simulink model "player_ball_7_8players2"  (R2021b)
settings: Solver=VariableStepAuto  StartTime=0.0  StopTime=300  RelTol=1e-3
model workspace (MAT data in the model file):
  trailfuzzy = 'trailfuzzy.fis'
values from neighbouring files (symbols this model uses):
  initBallPos = fieldCenter    [robotSoccerParams.m]
  robotDetectorMaxHits = 5    [robotSoccerParams.m]
  sampleTime = 0.05    [robotSoccerParams.m]
undefined symbols (not defined in the file or in its folder): DiscIntNeverNeededParam
libraries: mobileRoboticsLib x41, dspindex x13, fuzblock x8
(part 1 of 2)
settings Model: NumberOfSteps=10  Creator=kstkr  LastModifiedBy=kstkr
settings DebuggingCC: AlgebraicLoopMsg=none

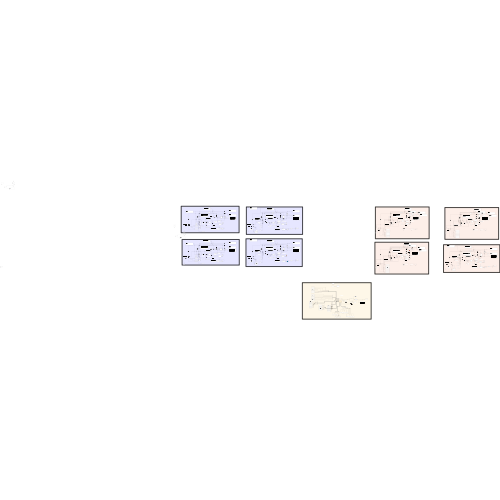
[thumbnail: Simulink's stored preview of the top-level diagram]
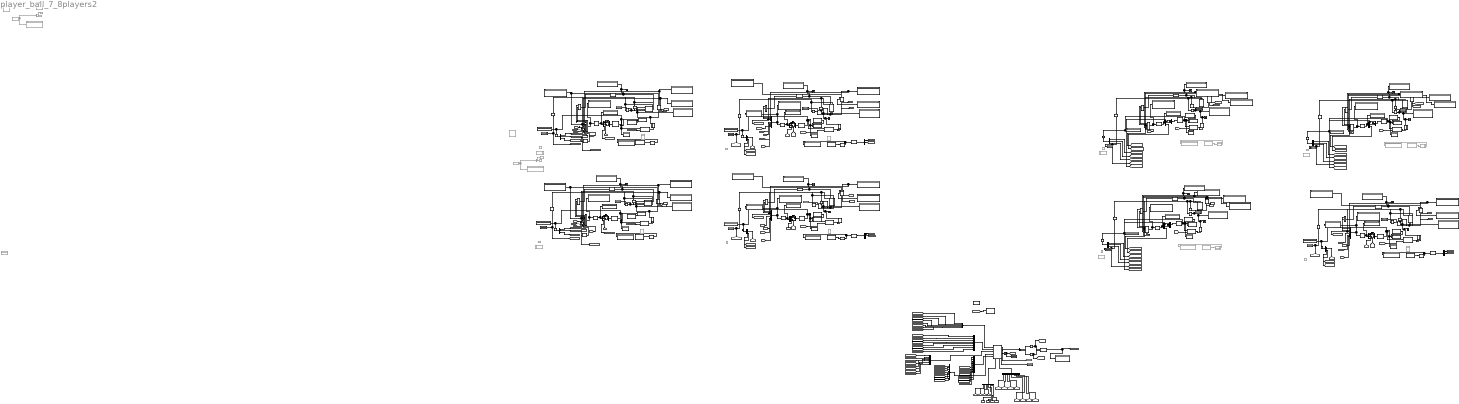
== system player_ball_7_8players2 ==
  note: Subsystem1
  note: Subsystem1
  note: Ensure the sensor parameters point to the same variables.
  note: Checks team possession and ball held
  note: change mf to sinesoidal
  note: check for postition 80,10
  note: Subsystem1
  note: change mf to sinesoidal
  note: check for postition 80,10
  note: Subsystem1
  note: Ensure the sensor parameters point to the same variables.
  note: Subsystem1
  note: Ensure the sensor parameters point to the same variables.
  note: Subsystem1
  note: Ensure the sensor parameters point to the same variables.
  note: Subsystem1
  note: Ensure the sensor parameters point to the same variables.
  note: Subsystem1
  note: Ensure the sensor parameters point to the same variables.
  Add Constant{,1..3} (4 alike) : Bias  Commented=on  Bias=0.3
  Ball Dynamics : MATLAB Function  Commented=on  TreatAsAtomicUnit=on
  Ball Dynamics1 : MATLAB Function  Commented=on  TreatAsAtomicUnit=on
  Ball Dynamics2 : MATLAB Function  Commented=on  TreatAsAtomicUnit=on
  Ball Dynamics3 : MATLAB Function  Commented=on  TreatAsAtomicUnit=on
  Ball Dynamics4 : MATLAB Function  Commented=on  TreatAsAtomicUnit=on
  Ball Dynamics5 : MATLAB Function  Commented=on  TreatAsAtomicUnit=on
  Ball Dynamics6 : MATLAB Function  Commented=on  TreatAsAtomicUnit=on
  Bus Creator{,1..6} (7 alike) : BusCreator  Inputs=8
  Chart3 : Stateflow chart  TreatAsAtomicUnit=on
      settings: PortSchema="{\"entries\":[{\"content\":{\"sides\":[{\"content\":{\"connectorIds\":[\"In1\",\"In2\",\"In3\",\"In4\",\"In6\"]},\"type\":\"ConnectorPlacement.EquallySpacedRectSide\",\"uuid\":\"100227f9-96df-4219-ace2-0d84d12d506e\"},{\"content\":{\"connectorIds\":[\"Out1\",\"Out2\",\"Out3\",\"Out4\"],\"side\":\"RIGHT\"},\"type\":\"ConnectorPlacement.EquallySpacedRectSide\",\"uuid\":\"5179a9f1-5caf-4bf7-8381-53191773d399\"},{\"content\":{\"connectorIds\":[],\"side\":\"TOP\"},\"type\":\"ConnectorPlacement.EquallySpacedRectSide\",\"uuid\":\"b02881a3-df96-4ac6-93d3-ffe2a0056366\"},{\"content\":{\"connectorIds\":[\"In7\",\"In5\"],\"side\":\"BOTTOM\"},\"type\":\"ConnectorPlacement.EquallySpacedRectSide\",\"uuid\":\"6df5f698-3dd3-4c11-801f-bca33302808b\"}]},\"type\":\"ConnectorPlacement.EquallySpacedConnector\",\"uuid\":\"a5fc3484-c51e-4d4d-931a-fb20b747c02a\"}],\"packageUris\":[\"http://schema.mathworks.com/mf0/Connector/R2020b\"],\"version\":\"1.0\"}"
  Constant{,1..8} (9 alike) : Constant  Commented=on  Value=0.5
  Demux{,1..3,5..10,12..24,26..29} (27 alike) : Demux  Outputs=3
  Demux11 : Demux  Outputs=2
  Demux25 : Demux  Commented=on  Outputs=2
  Demux4 : Demux  Commented=on  Outputs=2
  Display{,1..9,11..41,43..49,51..58,60..69,71..84,86..87} (82 alike) : Display
  Display{10,42,50,59,70} (5 alike) : Display  Commented=on
  Generic Vehicle Simulation : mobileRoboticsLib/Utilities/Generic Vehicle Simulation  initX=40  initY=10  initAngle=0  Ts=sampleTime
      settings: SourceProductName=Mobile Robotics Simulation Toolbox
  Generic Vehicle Simulation1 : mobileRoboticsLib/Utilities/Generic Vehicle Simulation  initX=30  initY=50  initAngle=0  Ts=sampleTime
      settings: SourceProductName=Mobile Robotics Simulation Toolbox
  Generic Vehicle Simulation2 : mobileRoboticsLib/Utilities/Generic Vehicle Simulation  initX=25  initY=30  initAngle=0  Ts=sampleTime
      settings: SourceProductName=Mobile Robotics Simulation Toolbox
  Generic Vehicle Simulation3 : mobileRoboticsLib/Utilities/Generic Vehicle Simulation  initX=2  initY=30  initAngle=0  Ts=sampleTime
      settings: SourceProductName=Mobile Robotics Simulation Toolbox
  Generic Vehicle Simulation4 : mobileRoboticsLib/Utilities/Generic Vehicle Simulation  initX=60  initY=40  initAngle=pi  Ts=sampleTime
      settings: SourceProductName=Mobile Robotics Simulation Library
  Generic Vehicle Simulation5 : mobileRoboticsLib/Utilities/Generic Vehicle Simulation  initX=60  initY=20  initAngle=pi  Ts=sampleTime
      settings: SourceProductName=Mobile Robotics Simulation Library
  Generic Vehicle Simulation6 : mobileRoboticsLib/Utilities/Generic Vehicle Simulation  initX=75  initY=30  initAngle=pi  Ts=sampleTime
      settings: SourceProductName=Mobile Robotics Simulation Library
  Generic Vehicle Simulation7 : mobileRoboticsLib/Utilities/Generic Vehicle Simulation  initX=88  initY=30  initAngle=pi  Ts=sampleTime
      settings: SourceProductName=Mobile Robotics Simulation Toolbox
  Goal Range{,1..4} (5 alike) : Display
  GoalLeftAngle{,1..4} (5 alike) : Display
  Ground{,1..7} (8 alike) : Ground
  IC{1,4,7,10,13,16,19,22} (8 alike) : InitialCondition
  IC{2..3,5..6,8..9,11..12,14..15,17..18,20..21,23..24} (16 alike) : InitialCondition  Value=0
  MATLAB Function : MATLAB Function  TreatAsAtomicUnit=on
  MATLAB Function1 : MATLAB Function  TreatAsAtomicUnit=on
  Memory{,2..4,7..10} (8 alike) : Memory  InitialCondition=[15 2 0]  InheritSampleTime=on
  Memory1 : Memory  InheritSampleTime=on
  Memory5 : Memory  InheritSampleTime=on  LinearizeAsDelay=on
  Memory6 : Memory  InheritSampleTime=on  LinearizeAsDelay=on
  Multi-Robot Environment : mobileRoboticsLib/Environments/Multi-Robot Environment  numRobots=8  mapName=map  showWaypoints=off  showObjects=on  objectColors=objColors  objectMarkers=objMarkers  showRobotIds=on  plotSensorLines=on
      settings: SourceProductName=Mobile Robotics Simulation Toolbox
  Multi-Robot Lidar Sensor1 : mobileRoboticsLib/Environments/Multi-Robot Lidar Sensor  robotIdx=1  mapName=map  sensorOffset=[0,0]  scanAngles=[-pi/4 0 pi/4]  maxRange=5
      settings: SourceProductName=Mobile Robotics Simulation Toolbox
  Multi-Robot Lidar Sensor2 : mobileRoboticsLib/Environments/Multi-Robot Lidar Sensor  robotIdx=2  mapName=map  sensorOffset=[0,0]  scanAngles=[-pi/4 0 pi/4]  maxRange=5
      settings: SourceProductName=Mobile Robotics Simulation Toolbox
  Multi-Robot Lidar Sensor3 : mobileRoboticsLib/Environments/Multi-Robot Lidar Sensor  robotIdx=3  mapName=map  sensorOffset=[0,0]  scanAngles=[-pi/4 0 pi/4]  maxRange=5
      settings: SourceProductName=Mobile Robotics Simulation Toolbox
  Multi-Robot Lidar Sensor4 : mobileRoboticsLib/Environments/Multi-Robot Lidar Sensor  robotIdx=4  mapName=map  sensorOffset=[0,0]  scanAngles=[-pi/4 0 pi/4]  maxRange=5
      settings: SourceProductName=Mobile Robotics Simulation Toolbox
  Multi-Robot Lidar Sensor5 : mobileRoboticsLib/Environments/Multi-Robot Lidar Sensor  robotIdx=5  mapName=map  sensorOffset=[0,0]  scanAngles=[-pi/4 0 pi/4]  maxRange=5
      settings: SourceProductName=Mobile Robotics Simulation Toolbox
  Multi-Robot Lidar Sensor6 : mobileRoboticsLib/Environments/Multi-Robot Lidar Sensor  robotIdx=6  mapName=map  sensorOffset=[0,0]  scanAngles=[-pi/4 0 pi/4]  maxRange=5
      settings: SourceProductName=Mobile Robotics Simulation Toolbox
  Multi-Robot Lidar Sensor7 : mobileRoboticsLib/Environments/Multi-Robot Lidar Sensor  robotIdx=7  mapName=map  sensorOffset=[0,0]  scanAngles=[-pi/4 0 pi/4]  maxRange=5
      settings: SourceProductName=Mobile Robotics Simulation Toolbox
  Multi-Robot Lidar Sensor8 : mobileRoboticsLib/Environments/Multi-Robot Lidar Sensor  robotIdx=8  mapName=map  sensorOffset=[0,0]  scanAngles=[-pi/4 0 pi/4]  maxRange=5
      settings: SourceProductName=Mobile Robotics Simulation Toolbox
  Multi-Robot Visualizer : mobileRoboticsLib/Environments/Multi-Robot Visualizer  idx=1  radius=1  robotColor=[0 0 1]  showTraj=on  hasLidar=on  sensorOffset=[0,0]  scanAngles=[-pi/4 0 pi/4]  maxNumScans=0  hasObjDetector=off  objDetectorOffset=[0,0]  objDetectorAngle=0  objDetectorFOV=pi/3  objDetectorMaxRange=5  hasRobotDetector=off  robotDetectorOffset=[0,0]  robotDetectorAngle=0  robotDetectorFOV=pi/3  robotDetectorMaxRange=5  robotDetectorNumDetections=0
      settings: SourceProductName=Mobile Robotics Simulation Toolbox
  Multi-Robot Visualizer1 : mobileRoboticsLib/Environments/Multi-Robot Visualizer  idx=3  radius=1  robotColor=[0 0 1]  showTraj=on  hasLidar=on  sensorOffset=[0,0]  scanAngles=[-pi/4 0 pi/4]  maxNumScans=0  hasObjDetector=off  objDetectorOffset=[0,0]  objDetectorAngle=0  objDetectorFOV=pi/3  objDetectorMaxRange=5  hasRobotDetector=off  robotDetectorOffset=[0,0]  robotDetectorAngle=0  robotDetectorFOV=pi/3  robotDetectorMaxRange=5  robotDetectorNumDetections=0
      settings: SourceProductName=Mobile Robotics Simulation Toolbox
  Multi-Robot Visualizer2 : mobileRoboticsLib/Environments/Multi-Robot Visualizer  idx=2  radius=1  robotColor=[0 0 1]  showTraj=on  hasLidar=on  sensorOffset=[0,0]  scanAngles=[-pi/4 0 pi/4]  maxNumScans=0  hasObjDetector=off  objDetectorOffset=[0,0]  objDetectorAngle=0  objDetectorFOV=pi/3  objDetectorMaxRange=5  hasRobotDetector=off  robotDetectorOffset=[0,0]  robotDetectorAngle=0  robotDetectorFOV=pi/3  robotDetectorMaxRange=5  robotDetectorNumDetections=0
      settings: SourceProductName=Mobile Robotics Simulation Toolbox
  Multi-Robot Visualizer3 : mobileRoboticsLib/Environments/Multi-Robot Visualizer  idx=4  radius=1  robotColor=[0 0 1]  showTraj=on  hasLidar=on  sensorOffset=[0,0]  scanAngles=[-pi/4 0 pi/4]  maxNumScans=0  hasObjDetector=off  objDetectorOffset=[0,0]  objDetectorAngle=0  objDetectorFOV=pi/3  objDetectorMaxRange=5  hasRobotDetector=off  robotDetectorOffset=[0,0]  robotDetectorAngle=0  robotDetectorFOV=pi/3  robotDetectorMaxRange=5  robotDetectorNumDetections=0
      settings: SourceProductName=Mobile Robotics Simulation Toolbox
  Multi-Robot Visualizer4 : mobileRoboticsLib/Environments/Multi-Robot Visualizer  idx=5  radius=1  robotColor=[1 0 0]  showTraj=on  hasLidar=on  sensorOffset=[0,0]  scanAngles=[-pi/4 0 pi/4]  maxNumScans=0  hasObjDetector=off  objDetectorOffset=[0,0]  objDetectorAngle=0  objDetectorFOV=pi/3  objDetectorMaxRange=5  hasRobotDetector=off  robotDetectorOffset=[0,0]  robotDetectorAngle=0  robotDetectorFOV=pi/3  robotDetectorMaxRange=5  robotDetectorNumDetections=0
      settings: SourceProductName=Mobile Robotics Simulation Toolbox
  Multi-Robot Visualizer5 : mobileRoboticsLib/Environments/Multi-Robot Visualizer  idx=6  radius=1  robotColor=[1 0 0]  showTraj=on  hasLidar=on  sensorOffset=[0,0]  scanAngles=[-pi/4 0 pi/4]  maxNumScans=0  hasObjDetector=off  objDetectorOffset=[0,0]  objDetectorAngle=0  objDetectorFOV=pi/3  objDetectorMaxRange=5  hasRobotDetector=off  robotDetectorOffset=[0,0]  robotDetectorAngle=0  robotDetectorFOV=pi/3  robotDetectorMaxRange=5  robotDetectorNumDetections=0
      settings: SourceProductName=Mobile Robotics Simulation Toolbox
  Multi-Robot Visualizer6 : mobileRoboticsLib/Environments/Multi-Robot Visualizer  idx=7  radius=1  robotColor=[1 0 0]  showTraj=on  hasLidar=on  sensorOffset=[0,0]  scanAngles=[-pi/4 0 pi/4]  maxNumScans=0  hasObjDetector=off  objDetectorOffset=[0,0]  objDetectorAngle=0  objDetectorFOV=pi/3  objDetectorMaxRange=5  hasRobotDetector=off  robotDetectorOffset=[0,0]  robotDetectorAngle=0  robotDetectorFOV=pi/3  robotDetectorMaxRange=5  robotDetectorNumDetections=0
      settings: SourceProductName=Mobile Robotics Simulation Toolbox
  Multi-Robot Visualizer7 : mobileRoboticsLib/Environments/Multi-Robot Visualizer  idx=8  radius=1  robotColor=[1 0 0]  showTraj=on  hasLidar=on  sensorOffset=[0,0]  scanAngles=[-pi/4 0 pi/4]  maxNumScans=0  hasObjDetector=off  objDetectorOffset=[0,0]  objDetectorAngle=0  objDetectorFOV=pi/3  objDetectorMaxRange=5  hasRobotDetector=off  robotDetectorOffset=[0,0]  robotDetectorAngle=0  robotDetectorFOV=pi/3  robotDetectorMaxRange=5  robotDetectorNumDetections=0
      settings: SourceProductName=Mobile Robotics Simulation Toolbox
  Mux{,1,4,6,8,10,12,14} (8 alike) : Mux  Inputs=3
  Mux11 : Mux  Inputs=7
  Mux13 : Mux  Inputs=7
  Mux15 : Mux  Inputs=8
  Mux2 : Mux  Inputs=11
  Mux3 : Mux  Inputs=11
  Mux5 : Mux  Inputs=9
  Mux7 : Mux  Inputs=8
  Mux9 : Mux  Inputs=7
  Object Detections [range, angle, label]{,1..7} (8 alike) : Display
  Object Detector{,1..7} (8 alike) : mobileRoboticsLib/Environments/Object Detector  mapName=map  sensorOffset=objDetectorOffset  sensorAngle=objDetectorAngle  fieldOfView=objDetectorFOV  maxRange=objDetectorRange  maxDetections=objDetectorMaxHits  sampleTime=-1
      Object Detector settings: SourceProductName=Mobile Robotics Simulation Toolbox
      Object Detector1 settings: SourceProductName=Mobile Robotics Simulation Toolbox
      Object Detector2 settings: SourceProductName=Mobile Robotics Simulation Toolbox
      Object Detector3 settings: SourceProductName=Mobile Robotics Simulation Toolbox
      Object Detector4 settings: SourceProductName=Ground Vehicles Library
      Object Detector5 settings: SourceProductName=Ground Vehicles Library
      Object Detector6 settings: SourceProductName=Ground Vehicles Library
      Object Detector7 settings: SourceProductName=Mobile Robotics Simulation Toolbox
  "Objects [x, y, label]1" : Constant  Commented=on  Value=[45, 30, 1; 0,15,2; 0, 45, 2; 90, 15, 3; 90, 45, 3]
  "Objects [x, y, label]2" : Constant  Commented=on  Value=[45, 30, 1; 0,15,2; 0, 45, 2; 90, 15, 3; 90, 45, 3]
  Package Objects Array1 : Subsystem
  Plot Soccer Field : MATLAB Function  TreatAsAtomicUnit=on
  Robot Detector1 : mobileRoboticsLib/Environments/Robot Detector  mapName=map  robotIdx=1  sensorOffset=robotDetectorOffset  sensorAngle=robotDetectorAngle  sensorFOV=2*pi  maxRange=100  maxDetections=robotDetectorMaxHits  sampleTime=sampleTime
      link override Robot Detector: mapName=map  maxDetections=5
      settings: SourceProductName=Mobile Robotics Simulation Toolbox
  Robot Detector2 : mobileRoboticsLib/Environments/Robot Detector  mapName=map  robotIdx=2  sensorOffset=robotDetectorOffset  sensorAngle=robotDetectorAngle  sensorFOV=2*pi  maxRange=100  maxDetections=robotDetectorMaxHits  sampleTime=sampleTime
      link override Robot Detector: mapName=map  maxDetections=5
      settings: SourceProductName=Mobile Robotics Simulation Toolbox
  Robot Detector3 : mobileRoboticsLib/Environments/Robot Detector  mapName=map  robotIdx=3  sensorOffset=robotDetectorOffset  sensorAngle=robotDetectorAngle  sensorFOV=2*pi  maxRange=100  maxDetections=robotDetectorMaxHits  sampleTime=sampleTime
      link override Robot Detector: mapName=map  maxDetections=5
      settings: SourceProductName=Mobile Robotics Simulation Toolbox
  Robot Detector4 : mobileRoboticsLib/Environments/Robot Detector  mapName=map  robotIdx=4  sensorOffset=robotDetectorOffset  sensorAngle=robotDetectorAngle  sensorFOV=2*pi  maxRange=100  maxDetections=robotDetectorMaxHits  sampleTime=sampleTime
      link override Robot Detector: mapName=map  maxDetections=5
      settings: SourceProductName=Mobile Robotics Simulation Toolbox
  Robot Detector5 : mobileRoboticsLib/Environments/Robot Detector  Commented=on  mapName=map  robotIdx=1  sensorOffset=robotDetectorOffset  sensorAngle=robotDetectorAngle  sensorFOV=pi/3  maxRange=100  maxDetections=robotDetectorMaxHits  sampleTime=sampleTime
      link override Robot Detector: mapName=map  maxDetections=5
      settings: SourceProductName=Mobile Robotics Simulation Toolbox
  Robot Detector6 : mobileRoboticsLib/Environments/Robot Detector  Commented=on  mapName=map  robotIdx=1  sensorOffset=robotDetectorOffset  sensorAngle=robotDetectorAngle  sensorFOV=pi/3  maxRange=100  maxDetections=robotDetectorMaxHits  sampleTime=sampleTime
      link override Robot Detector: mapName=map  maxDetections=5
      settings: SourceProductName=Mobile Robotics Simulation Toolbox
  Robot Detector7 : mobileRoboticsLib/Environments/Robot Detector  Commented=on  mapName=map  robotIdx=1  sensorOffset=robotDetectorOffset  sensorAngle=robotDetectorAngle  sensorFOV=pi/3  maxRange=100  maxDetections=robotDetectorMaxHits  sampleTime=sampleTime
      link override Robot Detector: mapName=map  maxDetections=5
      settings: SourceProductName=Mobile Robotics Simulation Toolbox
  Robot Detector8 : mobileRoboticsLib/Environments/Robot Detector  mapName=map  robotIdx=8  sensorOffset=robotDetectorOffset  sensorAngle=robotDetectorAngle  sensorFOV=2*pi  maxRange=100  maxDetections=robotDetectorMaxHits  sampleTime=sampleTime
      link override Robot Detector: mapName=map  maxDetections=5
      settings: SourceProductName=Mobile Robotics Simulation Toolbox
  Scope{,1..2,4,6,8,10,12} (8 alike) : Scope
  Scope{3,5,7,9,11,13} (6 alike) : Scope  NumInputPorts=2
  Variable Selector{,1,3..8,10..12} (11 alike) : dspindex/Variable Selector  NumInputs=1  rowsOrCols=Rows  IdxMode=Fixed  Elements="[1  ]"  ZerOneIdxMode=One-based  errmode=Clip Index  FillMode=off  FillValues=0
  Variable Selector2 : dspindex/Variable Selector  Commented=on  NumInputs=1  rowsOrCols=Columns  IdxMode=Fixed  Elements=[1 2]  ZerOneIdxMode=One-based  errmode=Clip Index  FillMode=on  FillValues=0
  Variable Selector9 : dspindex/Variable Selector  Commented=on  NumInputs=1  rowsOrCols=Columns  IdxMode=Fixed  Elements=[1 2]  ZerOneIdxMode=One-based  errmode=Clip Index  FillMode=on  FillValues=0
  Zero Pad Detections1 : MATLAB Function  TreatAsAtomicUnit=on  mask(Zero Pad Detections){maxHits=robotDetectorMaxHits}
      mask prompts: maxHits "Maximum Sensor Hits"
      mask help: Zero pads detections matrix so it is fixed-size and works with arrays of buses.
  Zero Pad Detections10 : MATLAB Function  TreatAsAtomicUnit=on  mask(Zero Pad Detections){maxHits=robotDetectorMaxHits}
      mask prompts: maxHits "Maximum Sensor Hits"
      mask help: Zero pads detections matrix so it is fixed-size and works with arrays of buses.
  Zero Pad Detections11 : MATLAB Function  Commented=on  TreatAsAtomicUnit=on  mask(Zero Pad Detections){maxHits=robotDetectorMaxHits}
      mask prompts: maxHits "Maximum Sensor Hits"
      mask help: Zero pads detections matrix so it is fixed-size and works with arrays of buses.
  Zero Pad Detections12 : MATLAB Function  TreatAsAtomicUnit=on  mask(Zero Pad Detections){maxHits=robotDetectorMaxHits}
      mask prompts: maxHits "Maximum Sensor Hits"
      mask help: Zero pads detections matrix so it is fixed-size and works with arrays of buses.
  Zero Pad Detections13 : MATLAB Function  Commented=on  TreatAsAtomicUnit=on  mask(Zero Pad Detections){maxHits=robotDetectorMaxHits}
      mask prompts: maxHits "Maximum Sensor Hits"
      mask help: Zero pads detections matrix so it is fixed-size and works with arrays of buses.
  Zero Pad Detections14 : MATLAB Function  Commented=on  TreatAsAtomicUnit=on  mask(Zero Pad Detections){maxHits=robotDetectorMaxHits}
      mask prompts: maxHits "Maximum Sensor Hits"
      mask help: Zero pads detections matrix so it is fixed-size and works with arrays of buses.
  Zero Pad Detections15 : MATLAB Function  TreatAsAtomicUnit=on  mask(Zero Pad Detections){maxHits=robotDetectorMaxHits}
      mask prompts: maxHits "Maximum Sensor Hits"
      mask help: Zero pads detections matrix so it is fixed-size and works with arrays of buses.
  Zero Pad Detections16 : MATLAB Function  TreatAsAtomicUnit=on  mask(Zero Pad Detections){maxHits=robotDetectorMaxHits}
      mask prompts: maxHits "Maximum Sensor Hits"
      mask help: Zero pads detections matrix so it is fixed-size and works with arrays of buses.
  Zero Pad Detections17 : MATLAB Function  Commented=on  TreatAsAtomicUnit=on  mask(Zero Pad Detections){maxHits=robotDetectorMaxHits}
      mask prompts: maxHits "Maximum Sensor Hits"
      mask help: Zero pads detections matrix so it is fixed-size and works with arrays of buses.
  Zero Pad Detections18 : MATLAB Function  TreatAsAtomicUnit=on  mask(Zero Pad Detections){maxHits=robotDetectorMaxHits}
      mask prompts: maxHits "Maximum Sensor Hits"
      mask help: Zero pads detections matrix so it is fixed-size and works with arrays of buses.
  Zero Pad Detections19 : MATLAB Function  TreatAsAtomicUnit=on  mask(Zero Pad Detections){maxHits=robotDetectorMaxHits}
      mask prompts: maxHits "Maximum Sensor Hits"
      mask help: Zero pads detections matrix so it is fixed-size and works with arrays of buses.
  Zero Pad Detections2 : MATLAB Function  TreatAsAtomicUnit=on  mask(Zero Pad Detections){maxHits=robotDetectorMaxHits}
      mask prompts: maxHits "Maximum Sensor Hits"
      mask help: Zero pads detections matrix so it is fixed-size and works with arrays of buses.
  Zero Pad Detections20 : MATLAB Function  Commented=on  TreatAsAtomicUnit=on  mask(Zero Pad Detections){maxHits=robotDetectorMaxHits}
      mask prompts: maxHits "Maximum Sensor Hits"
      mask help: Zero pads detections matrix so it is fixed-size and works with arrays of buses.
  Zero Pad Detections21 : MATLAB Function  TreatAsAtomicUnit=on  mask(Zero Pad Detections){maxHits=robotDetectorMaxHits}
      mask prompts: maxHits "Maximum Sensor Hits"
      mask help: Zero pads detections matrix so it is fixed-size and works with arrays of buses.
  Zero Pad Detections3 : MATLAB Function  Commented=on  TreatAsAtomicUnit=on  mask(Zero Pad Detections){maxHits=robotDetectorMaxHits}
      mask prompts: maxHits "Maximum Sensor Hits"
      mask help: Zero pads detections matrix so it is fixed-size and works with arrays of buses.
  Zero Pad Detections4 : MATLAB Function  TreatAsAtomicUnit=on  mask(Zero Pad Detections){maxHits=robotDetectorMaxHits}
      mask prompts: maxHits "Maximum Sensor Hits"
      mask help: Zero pads detections matrix so it is fixed-size and works with arrays of buses.
  Zero Pad Detections5 : MATLAB Function  TreatAsAtomicUnit=on  mask(Zero Pad Detections){maxHits=robotDetectorMaxHits}
      mask prompts: maxHits "Maximum Sensor Hits"
      mask help: Zero pads detections matrix so it is fixed-size and works with arrays of buses.
  Zero Pad Detections6 : MATLAB Function  Commented=on  TreatAsAtomicUnit=on  mask(Zero Pad Detections){maxHits=robotDetectorMaxHits}
      mask prompts: maxHits "Maximum Sensor Hits"
      mask help: Zero pads detections matrix so it is fixed-size and works with arrays of buses.
  Zero Pad Detections7 : MATLAB Function  TreatAsAtomicUnit=on  mask(Zero Pad Detections){maxHits=robotDetectorMaxHits}
      mask prompts: maxHits "Maximum Sensor Hits"
      mask help: Zero pads detections matrix so it is fixed-size and works with arrays of buses.
  Zero Pad Detections8 : MATLAB Function  Commented=on  TreatAsAtomicUnit=on  mask(Zero Pad Detections){maxHits=robotDetectorMaxHits}
      mask prompts: maxHits "Maximum Sensor Hits"
      mask help: Zero pads detections matrix so it is fixed-size and works with arrays of buses.
  Zero Pad Detections9 : MATLAB Function  TreatAsAtomicUnit=on  mask(Zero Pad Detections){maxHits=robotDetectorMaxHits}
      mask prompts: maxHits "Maximum Sensor Hits"
      mask help: Zero pads detections matrix so it is fixed-size and works with arrays of buses.
  ball : MATLAB Function  TreatAsAtomicUnit=on
  ball1 : MATLAB Function  TreatAsAtomicUnit=on
  ball2 : MATLAB Function  TreatAsAtomicUnit=on
  ball3 : MATLAB Function  TreatAsAtomicUnit=on
  ball4 : MATLAB Function  TreatAsAtomicUnit=on
  ball5 : MATLAB Function  TreatAsAtomicUnit=on
  ball6 : MATLAB Function  TreatAsAtomicUnit=on
  ball7 : MATLAB Function  TreatAsAtomicUnit=on
  idx3 goal_range_angles : MATLAB Function  TreatAsAtomicUnit=on
  idx3 goal_range_angles1 : MATLAB Function  TreatAsAtomicUnit=on
  idx3 goal_range_angles2 : MATLAB Function  TreatAsAtomicUnit=on
  idx3 goal_range_angles3 : MATLAB Function  TreatAsAtomicUnit=on
  idx3 goal_range_angles4 : MATLAB Function  TreatAsAtomicUnit=on
  idx3 goal_range_angles5 : MATLAB Function  TreatAsAtomicUnit=on
  idx3 goal_range_angles6 : MATLAB Function  TreatAsAtomicUnit=on
  idx3 goal_range_angles7 : MATLAB Function  TreatAsAtomicUnit=on
  robot_actions1 : fuzblock/Fuzzy Logic  Controller  FIS='A1trialfuzzyball8L.fis'  OutputSampleNumber=101  DataType=double  FuzzifiedInputs=off  RuleFiringStrengths=off  RuleOutputs=off  AggregatedOutputs=off  SimulateUsing=Interpreted execution  OutOfRangeInputValueMessage=warning  NoRuleFiredMessage=warning  EmptyOutputFuzzySetMessage=warning
  robot_actions2 : fuzblock/Fuzzy Logic  Controller  FIS='A1trialfuzzyball8U.fis'  OutputSampleNumber=101  DataType=double  FuzzifiedInputs=off  RuleFiringStrengths=off  RuleOutputs=off  AggregatedOutputs=off  SimulateUsing=Interpreted execution  OutOfRangeInputValueMessage=warning  NoRuleFiredMessage=warning  EmptyOutputFuzzySetMessage=warning
  robot_actions3 : fuzblock/Fuzzy Logic  Controller  FIS='D1trialfuzzyball6.fis'  OutputSampleNumber=101  DataType=double  FuzzifiedInputs=off  RuleFiringStrengths=off  RuleOutputs=off  AggregatedOutputs=off  SimulateUsing=Interpreted execution  OutOfRangeInputValueMessage=warning  NoRuleFiredMessage=warning  EmptyOutputFuzzySetMessage=warning
  robot_actions4 : fuzblock/Fuzzy Logic  Controller  FIS='G1trialfuzzyball4.fis'  OutputSampleNumber=101  DataType=double  FuzzifiedInputs=off  RuleFiringStrengths=off  RuleOutputs=off  AggregatedOutputs=off  SimulateUsing=Interpreted execution  OutOfRangeInputValueMessage=warning  NoRuleFiredMessage=warning  EmptyOutputFuzzySetMessage=warning
  robot_actions5 : fuzblock/Fuzzy Logic  Controller  FIS='A1trialfuzzyball3.fis'  OutputSampleNumber=101  DataType=double  FuzzifiedInputs=off  RuleFiringStrengths=off  RuleOutputs=off  AggregatedOutputs=off  SimulateUsing=Interpreted execution  OutOfRangeInputValueMessage=warning  NoRuleFiredMessage=warning  EmptyOutputFuzzySetMessage=warning
  robot_actions6 : fuzblock/Fuzzy Logic  Controller  FIS='A1trialfuzzyball3.fis'  OutputSampleNumber=101  DataType=double  FuzzifiedInputs=off  RuleFiringStrengths=off  RuleOutputs=off  AggregatedOutputs=off  SimulateUsing=Interpreted execution  OutOfRangeInputValueMessage=warning  NoRuleFiredMessage=warning  EmptyOutputFuzzySetMessage=warning
  robot_actions7 : fuzblock/Fuzzy Logic  Controller  FIS='A1trialfuzzyball3.fis'  OutputSampleNumber=101  DataType=double  FuzzifiedInputs=off  RuleFiringStrengths=off  RuleOutputs=off  AggregatedOutputs=off  SimulateUsing=Interpreted execution  OutOfRangeInputValueMessage=warning  NoRuleFiredMessage=warning  EmptyOutputFuzzySetMessage=warning
  robot_actions8 : fuzblock/Fuzzy Logic  Controller  FIS='G2trialfuzzyball4.fis'  OutputSampleNumber=101  DataType=double  FuzzifiedInputs=off  RuleFiringStrengths=off  RuleOutputs=off  AggregatedOutputs=off  SimulateUsing=Interpreted execution  OutOfRangeInputValueMessage=warning  NoRuleFiredMessage=warning  EmptyOutputFuzzySetMessage=warning
  wires:
  Robot Detector1/1 -> Zero Pad Detections2/1(u)
  Zero Pad Detections2/1(y) -> Display5/1  "robotDetections"
  Mux/1 -> Generic Vehicle Simulation/1
  Ground/1 -> Mux/2
  robot_actions1/1 -> Display13/1, Demux/1  "v"
  Demux/1 -> [ballVel1], Mux/1
  Demux/2 -> Mux/3
  Generic Vehicle Simulation/1 -> Display11/1, Memory/1, Display/1, Object Detector/1, Multi-Robot Visualizer/1  "pose"
  Mux2/1 -> Display3/1, robot_actions1/1
  Object Detector/1 -> Zero Pad Detections4/1(u)  "detections"
  Variable Selector/1 -> Demux2/1
  Demux2/1 -> Mux2/2
  Multi-Robot Lidar Sensor1/1 -> Multi-Robot Visualizer/2
  [objPoses] -> Multi-Robot Environment/1
  Demux2/2 -> Mux2/1
  Zero Pad Detections4/1(y) -> ball/1(u), "Object Detections [range, angle, label]"/1, idx3 goal_range_angles/1(u)  "robotDetections"
  ball/1(y) -> Scope/1, Display9/1, Variable Selector/1
  idx3 goal_range_angles/1(goalRight_angle) -> Mux2/4, Display6/1
  idx3 goal_range_angles/2(goalRange) -> Goal Range/1, Mux2/5
  idx3 goal_range_angles/3(goalLeft_angle) -> Mux2/6, GoalLeftAngle/1
  Variable Selector2/1 -> Demux4/1, Display10/1
  Demux4/1 -> Add Constant/1
  Demux4/2 -> Add Constant1/1
  Memory/1 -> Demux6/1
  Demux6/1 -> [rPose_x1]
  Demux6/2 -> [rPose_y1]
  Demux6/3 -> [rPose_theta1]
  Demux/3 -> [KickPower1]
  ball/3(robotIdx) -> IC1/1, IC2/1
  IC1/1 -> [robotIdx1], Display15/1
  ball/2(ballHeld) -> [ballHeld1], Mux2/3, IC3/1
  IC2/1 -> Display14/1, ball/3("robotIdx ")
  IC3/1 -> ball/2("ballHeld ")
  IC6/1 -> Display18/1, ball1/2("ballHeld ")
  IC5/1 -> ball1/3("robotIdx ")
  ball1/2(ballHeld) -> IC6/1, [ballHeld2], Mux5/3
  IC4/1 -> Display19/1, [robotIdx2]
  ball1/3(robotIdx) -> IC5/1, IC4/1
  Demux7/3 -> [KickPower2]
  Demux10/3 -> [rPose_theta2]
  Demux10/2 -> [rPose_y2]
  Demux10/1 -> [rPose_x2]
  Memory4/1 -> Demux10/1
  idx3 goal_range_angles1/3(goalLeft_angle) -> GoalLeftAngle1/1
  idx3 goal_range_angles1/2(goalRange) -> Mux5/4, Goal Range1/1
  idx3 goal_range_angles1/1(goalRight_angle) -> Display22/1
  ball1/1(y) -> Variable Selector3/1, Display23/1, Scope1/1
  Zero Pad Detections7/1(y) -> "Object Detections [range, angle, label]2"/1, ball1/1(u), idx3 goal_range_angles1/1(u), Scope3/1  "robotDetections"
  Demux8/2 -> Mux5/1
  Multi-Robot Lidar Sensor2/1 -> Multi-Robot Visualizer2/2
  Demux8/1 -> Mux5/2
  Variable Selector3/1 -> Demux8/1
  Object Detector2/1 -> Zero Pad Detections7/1(u)  "detections"
  Mux5/1 -> robot_actions3/1, Display16/1, Display20/1
  Generic Vehicle Simulation2/1 -> Multi-Robot Visualizer2/1, Display7/1, Object Detector2/1, Memory4/1, Display8/1  "pose"
  Demux7/2 -> Mux4/3
  Demux7/1 -> [ballVel2], Mux4/1
  robot_actions3/1 -> Demux7/1, Display17/1  "v"
  Ground2/1 -> Mux4/2
  Mux4/1 -> Generic Vehicle Simulation2/1
  Zero Pad Detections5/1(y) -> Variable Selector4/1, Display21/1  "robotDetections"
  Robot Detector2/1 -> Zero Pad Detections5/1(u)
  [objPoses] -> Object Detector/2
  [objPoses] -> Object Detector2/2
  Demux9/2 -> [rdet_angle]
  Demux9/1 -> [rdet_range]
  [rdet_range] -> Mux5/5
  [rdet_angle] -> Mux5/6
  Variable Selector4/1 -> Demux9/1
  Chart3/1(ballPose) -> Demux11/1
  [rPose_theta2] -> Bus Creator6/2
  [rPose_theta1] -> Bus Creator6/1
  [ballVel2] -> Bus Creator5/2
  [ballVel1] -> Bus Creator5/1
  [robotIdx2] -> Bus Creator2/2
  [robotIdx1] -> Bus Creator2/1
  [rPose_y2] -> Bus Creator4/2
  [rPose_y1] -> Bus Creator4/1
  [rPose_x2] -> Bus Creator3/2
  [rPose_x1] -> Bus Creator3/1
  [KickPower2] -> Bus Creator1/2
  [KickPower1] -> Bus Creator1/1
  [ballHeld2] -> Bus Creator/2
  [ballHeld1] -> Bus Creator/1
  Bus Creator6/1 -> Chart3/5(rPose_theta)
  Bus Creator5/1 -> Chart3/7(ballVel)
  Bus Creator4/1 -> Chart3/4(rPose_y)
  Bus Creator3/1 -> Chart3/3(rPose_x)
  Bus Creator2/1 -> Chart3/6(robotIdx)
  Bus Creator1/1 -> Chart3/2(KickPower)
  Bus Creator/1 -> Chart3/1(ballHeld)
  Package Objects Array1/1(objectsPose) -> Display24/1, [objPoses]
  Memory5/1 -> [ballPose_y], Package Objects Array1/2(In2)
  Memory6/1 -> [ballPose_x], Package Objects Array1/1(Inport)
  Demux11/2 -> Memory5/1
  Demux11/1 -> Memory6/1
  Chart3/2(teamHeld) -> Memory1/1
  [ballPose_x] -> Mux5/7
  [teamHeld] -> Mux5/8
  Memory1/1 -> Display1/1, [teamHeld]
  [teamHeld] -> Mux2/7
  [rPose_x1] -> Mux2/8
  [rPose_x1] -> idx3 goal_range_angles/2(rPose_x)
  [rPose_y1] -> idx3 goal_range_angles/3(rPose_y)
  [rPose_x2] -> idx3 goal_range_angles1/2(rPose_x)
  [rPose_y2] -> idx3 goal_range_angles1/3(rPose_y)
  [rPose_theta1] -> MATLAB Function/1(u)
  [rPose_y1] -> Mux2/10
  MATLAB Function/1(y) -> Mux2/9
  MATLAB Function1/1(y) -> Mux3/9
  [rPose_y3] -> Mux3/10
  [rPose_theta3] -> MATLAB Function1/1(u)
  [rPose_y3] -> idx3 goal_range_angles3/3(rPose_y)
  [rPose_x3] -> idx3 goal_range_angles3/2(rPose_x)
  [rPose_x3] -> Mux3/8
  [teamHeld] -> Mux3/7
  [objPoses] -> Object Detector1/2
  IC9/1 -> ball3/2("ballHeld ")
  IC8/1 -> ball3/3("robotIdx "), Display25/1
  ball3/2(ballHeld) -> IC9/1, Mux3/3, [ballHeld3]
  IC7/1 -> Display26/1, [robotIdx3]
  ball3/3(robotIdx) -> IC8/1, IC7/1
  Demux1/3 -> [KickPower3]
  Demux5/3 -> [rPose_theta3]
  Demux5/2 -> [rPose_y3]
  Demux5/1 -> [rPose_x3]
  Memory2/1 -> Demux5/1
  idx3 goal_range_angles3/3(goalLeft_angle) -> GoalLeftAngle2/1, Mux3/6
  idx3 goal_range_angles3/2(goalRange) -> Mux3/5, Goal Range2/1
  idx3 goal_range_angles3/1(goalRight_angle) -> Display29/1, Mux3/4
  ball3/1(y) -> Variable Selector1/1, Display30/1, Scope2/1
  Zero Pad Detections9/1(y) -> idx3 goal_range_angles3/1(u), "Object Detections [range, angle, label]1"/1, ball3/1(u)  "robotDetections"
  Demux3/2 -> Mux3/1
  Multi-Robot Lidar Sensor3/1 -> Multi-Robot Visualizer1/2
  Demux3/1 -> Mux3/2
  Variable Selector1/1 -> Demux3/1
  Object Detector1/1 -> Zero Pad Detections9/1(u)  "detections"
  Mux3/1 -> robot_actions2/1, Display27/1
  Generic Vehicle Simulation1/1 -> Multi-Robot Visualizer1/1, Object Detector1/1, Display2/1, Memory2/1, Display4/1  "pose"
  Demux1/2 -> Mux1/3
  Demux1/1 -> Mux1/1, [ballVel3]
  robot_actions2/1 -> Demux1/1, Display12/1  "v"
  Ground1/1 -> Mux1/2
  Mux1/1 -> Generic Vehicle Simulation1/1
  Zero Pad Detections1/1(y) -> Display28/1  "robotDetections"
  Robot Detector3/1 -> Zero Pad Detections1/1(u)
  [rPose_y4] -> idx3 goal_range_angles4/3(rPose_y)
  [rPose_x4] -> idx3 goal_range_angles4/2(rPose_x)
  [teamHeld] -> Mux7/8
  [ballPose_x] -> Mux7/7
  Variable Selector6/1 -> Demux15/1
  [rdet_angle2] -> Mux7/6
  [rdet_range2] -> Mux7/5
  Demux15/1 -> [rdet_range2]
  Demux15/2 -> [rdet_angle2]
  [objPoses] -> Object Detector3/2
  Robot Detector4/1 -> Zero Pad Detections10/1(u)
  Zero Pad Detections10/1(y) -> Display36/1, Variable Selector6/1  "robotDetections"
  Mux6/1 -> Generic Vehicle Simulation3/1
  Ground3/1 -> Mux6/2
  robot_actions4/1 -> Display32/1, Demux13/1  "v"
  Demux13/1 -> Mux6/1, [ballVel4]
  Demux13/2 -> Mux6/3
  Generic Vehicle Simulation3/1 -> Display40/1, Memory3/1, Object Detector3/1, Display39/1, Multi-Robot Visualizer3/1  "pose"
  Mux7/1 -> Display35/1, Display31/1, robot_actions4/1
  Object Detector3/1 -> Zero Pad Detections12/1(u)  "detections"
  Variable Selector5/1 -> Demux14/1
  Demux14/1 -> Mux7/2
  Multi-Robot Lidar Sensor4/1 -> Multi-Robot Visualizer3/2
  Demux14/2 -> Mux7/1
  Zero Pad Detections12/1(y) -> Scope5/1, idx3 goal_range_angles4/1(u), ball4/1(u), "Object Detections [range, angle, label]3"/1  "robotDetections"
  ball4/1(y) -> Scope4/1, Display38/1, Variable Selector5/1
  idx3 goal_range_angles4/1(goalRight_angle) -> Display37/1
  idx3 goal_range_angles4/2(goalRange) -> Goal Range3/1, Mux7/4
  idx3 goal_range_angles4/3(goalLeft_angle) -> GoalLeftAngle3/1
  Memory3/1 -> Demux12/1
  Demux12/1 -> [rPose_x4]
  Demux12/2 -> [rPose_y4]
  Demux12/3 -> [rPose_theta4]
  Demux13/3 -> [KickPower4]
  ball4/3(robotIdx) -> IC10/1, IC11/1
  IC10/1 -> [robotIdx4], Display34/1
  ball4/2(ballHeld) -> Mux7/3, [ballHeld4], IC12/1
  IC11/1 -> ball4/3("robotIdx ")
  IC12/1 -> ball4/2("ballHeld "), Display33/1
  [ballHeld3] -> Bus Creator/3
  [ballHeld4] -> Bus Creator/4
  [KickPower3] -> Bus Creator1/3
  [KickPower4] -> Bus Creator1/4
  [rPose_x3] -> Bus Creator3/3
  [rPose_x4] -> Bus Creator3/4
  [rPose_y3] -> Bus Creator4/3
  [rPose_y4] -> Bus Creator4/4
  [robotIdx3] -> Bus Creator2/3
  [robotIdx4] -> Bus Creator2/4
  [ballVel3] -> Bus Creator5/3
  [ballVel4] -> Bus Creator5/4
  [rPose_theta3] -> Bus Creator6/3
  [rPose_theta4] -> Bus Creator6/4
  Demux25/2 -> Add Constant3/1
  Demux25/1 -> Add Constant2/1
  Variable Selector9/1 -> Display42/1, Demux25/1
  [ballHeld5] -> Bus Creator/5
  [ballHeld6] -> Bus Creator/6
  [ballHeld7] -> Bus Creator/7
  [ballHeld8] -> Bus Creator/8
  [KickPower8] -> Bus Creator1/8
  [KickPower7] -> Bus Creator1/7
  [KickPower5] -> Bus Creator1/5
  [KickPower6] -> Bus Creator1/6
  [rPose_x8] -> Bus Creator3/8
  [rPose_x7] -> Bus Creator3/7
  [rPose_x5] -> Bus Creator3/5
  [rPose_x6] -> Bus Creator3/6
  [rPose_y5] -> Bus Creator4/5
  [rPose_y6] -> Bus Creator4/6
  [rPose_y7] -> Bus Creator4/7
  [rPose_y8] -> Bus Creator4/8
  [robotIdx5] -> Bus Creator2/5
  [robotIdx6] -> Bus Creator2/6
  [robotIdx7] -> Bus Creator2/7
  [robotIdx8] -> Bus Creator2/8
  [ballVel8] -> Bus Creator5/8
  [ballVel7] -> Bus Creator5/7
  [ballVel5] -> Bus Creator5/5
  [ballVel6] -> Bus Creator5/6
  [rPose_theta8] -> Bus Creator6/8
  [rPose_theta7] -> Bus Creator6/7
  [rPose_theta5] -> Bus Creator6/5
  [rPose_theta6] -> Bus Creator6/6
  IC15/1 -> ball2/2("ballHeld ")
  IC14/1 -> ball2/3("robotIdx "), Display47/1
  ball2/2(ballHeld) -> [ballHeld5], Mux9/3, IC15/1
  IC13/1 -> [robotIdx5], Display48/1
  ball2/3(robotIdx) -> IC13/1, IC14/1
  Demux16/3 -> [KickPower5]
  Demux20/3 -> [rPose_theta5]
  Demux20/2 -> [rPose_y5]
  Demux20/1 -> [rPose_x5]
  Memory7/1 -> Demux20/1
  idx3 goal_range_angles2/3(goalLeft_angle) -> Mux9/6, Display53/1
  idx3 goal_range_angles2/2(goalRange) -> Mux9/5, Display52/1
  idx3 goal_range_angles2/1(goalRight_angle) -> Display51/1, Mux9/4
  ball2/1(y) -> Variable Selector7/1, Display54/1, Scope6/1
  Zero Pad Detections15/1(y) -> ball2/1(u), idx3 goal_range_angles2/1(u), "Object Detections [range, angle, label]4"/1, Scope7/1  "robotDetections"
  Demux17/2 -> Mux9/1
  Multi-Robot Lidar Sensor5/1 -> Multi-Robot Visualizer4/2
  Demux17/1 -> Mux9/2
  Variable Selector7/1 -> Demux17/1
  Object Detector4/1 -> Zero Pad Detections15/1(u)  "detections"
  Mux9/1 -> robot_actions5/1, Display49/1
  Generic Vehicle Simulation4/1 -> Multi-Robot Visualizer4/1, Display41/1, Object Detector4/1, Display44/1, Memory7/1  "pose"
  Demux16/2 -> Mux8/3
  Demux16/1 -> [ballVel5], Mux8/1
  robot_actions5/1 -> Demux16/1, Display46/1  "v"
  Ground4/1 -> Mux8/2
  Mux8/1 -> Generic Vehicle Simulation4/1
  Zero Pad Detections13/1(y) -> Display50/1  "robotDetections"
  Robot Detector5/1 -> Zero Pad Detections13/1(u)
  [objPoses] -> Object Detector4/2
  [objPoses] -> Object Detector5/2
  Robot Detector6/1 -> Zero Pad Detections14/1(u)
  Zero Pad Detections14/1(y) -> Display59/1  "robotDetections"
  Mux10/1 -> Generic Vehicle Simulation5/1
  Ground5/1 -> Mux10/2
  robot_actions6/1 -> Display55/1, Demux18/1  "v"
  Demux18/1 -> Mux10/1, [ballVel6]
  Demux18/2 -> Mux10/3
  Generic Vehicle Simulation5/1 -> Memory8/1, Display45/1, Object Detector5/1, Display43/1, Multi-Robot Visualizer5/1  "pose"
  Mux11/1 -> Display58/1, robot_actions6/1
  Object Detector5/1 -> Zero Pad Detections16/1(u)  "detections"
  Variable Selector8/1 -> Demux19/1
  Demux19/1 -> Mux11/2
  Multi-Robot Lidar Sensor6/1 -> Multi-Robot Visualizer5/2
  Demux19/2 -> Mux11/1
  Zero Pad Detections16/1(y) -> Scope9/1, "Object Detections [range, angle, label]5"/1, idx3 goal_range_angles5/1(u), ball5/1(u)  "robotDetections"
  ball5/1(y) -> Scope8/1, Display63/1, Variable Selector8/1
  idx3 goal_range_angles5/1(goalRight_angle) -> Mux11/4, Display60/1
  idx3 goal_range_angles5/2(goalRange) -> Mux11/5, Display61/1
  idx3 goal_range_angles5/3(goalLeft_angle) -> Mux11/6, Display62/1
  Memory8/1 -> Demux21/1
  Demux21/1 -> [rPose_x6]
  Demux21/2 -> [rPose_y6]
  Demux21/3 -> [rPose_theta6]
  Demux18/3 -> [KickPower6]
  ball5/3(robotIdx) -> IC17/1, IC16/1
  IC16/1 -> Display57/1, [robotIdx6]
  ball5/2(ballHeld) -> IC18/1, Mux11/3, [ballHeld6]
  IC17/1 -> Display56/1, ball5/3("robotIdx ")
  IC18/1 -> ball5/2("ballHeld ")
  [objPoses] -> Object Detector6/2
  Robot Detector7/1 -> Zero Pad Detections17/1(u)
  Zero Pad Detections17/1(y) -> Display70/1  "robotDetections"
  Mux12/1 -> Generic Vehicle Simulation6/1
  Ground6/1 -> Mux12/2
  robot_actions7/1 -> Display66/1, Demux22/1  "v"
  Demux22/1 -> Mux12/1, [ballVel7]
  Demux22/2 -> Mux12/3
  Generic Vehicle Simulation6/1 -> Memory9/1, Display65/1, Object Detector6/1, Display64/1, Multi-Robot Visualizer6/1  "pose"
  Mux13/1 -> Display69/1, robot_actions7/1
  Object Detector6/1 -> Zero Pad Detections18/1(u)  "detections"
  Variable Selector10/1 -> Demux23/1
  Demux23/1 -> Mux13/2
  Multi-Robot Lidar Sensor7/1 -> Multi-Robot Visualizer6/2
  Demux23/2 -> Mux13/1
  Zero Pad Detections18/1(y) -> Scope11/1, "Object Detections [range, angle, label]6"/1, idx3 goal_range_angles6/1(u), ball6/1(u)  "robotDetections"
  ball6/1(y) -> Scope10/1, Display74/1, Variable Selector10/1
  idx3 goal_range_angles6/1(goalRight_angle) -> Mux13/4, Display71/1
  idx3 goal_range_angles6/2(goalRange) -> Mux13/5, Display72/1
  idx3 goal_range_angles6/3(goalLeft_angle) -> Mux13/6, Display73/1
  Memory9/1 -> Demux24/1
  Demux24/1 -> [rPose_x7]
  Demux24/2 -> [rPose_y7]
  Demux24/3 -> [rPose_theta7]
  Demux22/3 -> [KickPower7]
  ball6/3(robotIdx) -> IC20/1, IC19/1
  IC19/1 -> Display68/1, [robotIdx7]
  ball6/2(ballHeld) -> IC21/1, Mux13/3, [ballHeld7]
  IC20/1 -> Display67/1, ball6/3("robotIdx ")
  IC21/1 -> ball6/2("ballHeld ")
  [rPose_x5] -> idx3 goal_range_angles2/2(rPose_x)
  [rPose_y5] -> idx3 goal_range_angles2/3(rPose_y)
  [rPose_x6] -> idx3 goal_range_angles5/2(rPose_x)
  [rPose_y6] -> idx3 goal_range_angles5/3(rPose_y)
  [rPose_x7] -> idx3 goal_range_angles6/2(rPose_x)
  [rPose_y7] -> idx3 goal_range_angles6/3(rPose_y)
  Chart3/3(Team1score) -> Display86/1
  Chart3/4(Team2score) -> Display87/1
  IC24/1 -> Display77/1, ball7/2("ballHeld ")
  IC23/1 -> ball7/3("robotIdx ")
  ball7/2(ballHeld) -> IC24/1, [ballHeld8], Mux15/3
  IC22/1 -> Display78/1, [robotIdx8]
  ball7/3(robotIdx) -> IC23/1, IC22/1
  Demux27/3 -> [KickPower8]
  Demux26/3 -> [rPose_theta8]
  Demux26/2 -> [rPose_y8]
  Demux26/1 -> [rPose_x8]
  Memory10/1 -> Demux26/1
  idx3 goal_range_angles7/3(goalLeft_angle) -> GoalLeftAngle4/1
  idx3 goal_range_angles7/2(goalRange) -> Mux15/4, Goal Range4/1
  idx3 goal_range_angles7/1(goalRight_angle) -> Display81/1
  ball7/1(y) -> Variable Selector11/1, Display82/1, Scope12/1
  Zero Pad Detections21/1(y) -> "Object Detections [range, angle, label]7"/1, ball7/1(u), idx3 goal_range_angles7/1(u), Scope13/1  "robotDetections"
  Demux28/2 -> Mux15/1
  Multi-Robot Lidar Sensor8/1 -> Multi-Robot Visualizer7/2
  Demux28/1 -> Mux15/2
  Variable Selector11/1 -> Demux28/1
  Object Detector7/1 -> Zero Pad Detections21/1(u)  "detections"
  Mux15/1 -> robot_actions8/1, Display75/1, Display79/1
  Generic Vehicle Simulation7/1 -> Multi-Robot Visualizer7/1, Display83/1, Object Detector7/1, Memory10/1, Display84/1  "pose"
  Demux27/2 -> Mux14/3
  Demux27/1 -> [ballVel8], Mux14/1
  robot_actions8/1 -> Demux27/1, Display76/1  "v"
  Ground7/1 -> Mux14/2
  Mux14/1 -> Generic Vehicle Simulation7/1
  Zero Pad Detections19/1(y) -> Variable Selector12/1, Display80/1  "robotDetections"
  Robot Detector8/1 -> Zero Pad Detections19/1(u)
  [objPoses] -> Object Detector7/2
  Demux29/2 -> [rdet_angle8]
  Demux29/1 -> [rdet_range8]
  [rdet_range8] -> Mux15/5
  [rdet_angle8] -> Mux15/6
  Variable Selector12/1 -> Demux29/1
  [ballPose_x] -> Mux15/7
  [teamHeld] -> Mux15/8
  [rPose_x4] -> idx3 goal_range_angles7/2(rPose_x)
  [rPose_y4] -> idx3 goal_range_angles7/3(rPose_y)
  [ballPose_y] -> Mux2/11
  [ballPose_y] -> Mux3/11
  [rPose_theta2] -> Mux5/9
  [teamHeld] -> Mux9/7
  [teamHeld] -> Mux11/7
  [teamHeld] -> Mux13/7

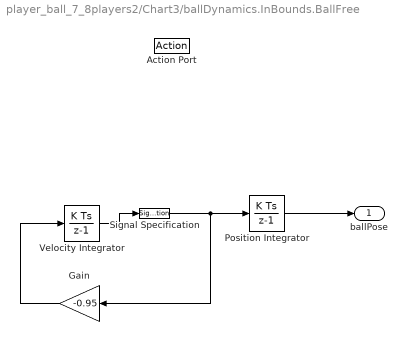
== system player_ball_7_8players2/Chart3/ballDynamics.InBounds.BallFree ==
  Action Port : ActionPort
      settings: CopyFcn=Stateflow.SLINSF.SimulinkMan.removeBlockPreDeleteFcn  PreDeleteFcn=Stateflow.SLINSF.SimulinkMan.unsafePredeleteFcn
  Gain : Gain  Gain=-0.95
  Position Integrator : DiscreteIntegrator  InitialCondition=initBallPos  SampleTime=-1  StateName=ballPos  ICPrevOutput=DiscIntNeverNeededParam  ICPrevScaledInput=DiscIntNeverNeededParam
  Signal Specification : SignalSpecification  Dimensions=[1 2]
  Velocity Integrator : DiscreteIntegrator  InitialCondition=[0 0]  SampleTime=-1  StateName=ballVel  ICPrevOutput=DiscIntNeverNeededParam  ICPrevScaledInput=DiscIntNeverNeededParam
  ballPose : Outport  VectorParamsAs1DForOutWhenUnconnected=off
  wires:
  Gain/1 -> Velocity Integrator/1
  Velocity Integrator/1 -> Signal Specification/1
  Position Integrator/1 -> ballPose/1
  Signal Specification/1 -> Position Integrator/1, Gain/1

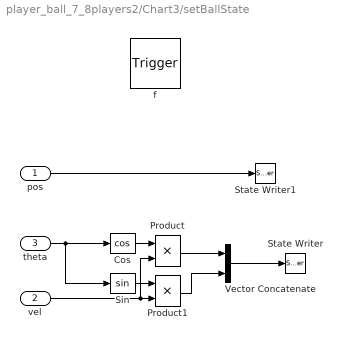
== system player_ball_7_8players2/Chart3/setBallState ==
  pos : Inport  OutDataTypeStr=double  PortDimensions=[1 2]
  vel : Inport  Port=2  OutDataTypeStr=double  PortDimensions=1
  theta : Inport  Port=3  OutDataTypeStr=double  PortDimensions=1
  f : TriggerPort  TriggerType=function-call  VariantControl=(inherit)
      settings: CopyFcn=Stateflow.SLINSF.SimulinkMan.removeBlockPreDeleteFcn  PreDeleteFcn=Stateflow.SLINSF.SimulinkMan.unsafePredeleteFcn
  Cos : Trigonometry  Operator=cos
  Product : Product
  Product1 : Product
  Sin : Trigonometry
  State Writer : StateWriter  StateOwnerBlock=../../ballDynamics.InBounds.BallFree/Velocity Integrator  StateName=ballVel
  State Writer1 : StateWriter  StateOwnerBlock=../../ballDynamics.InBounds.BallFree/Position Integrator  StateName=ballPos
  Vector Concatenate : Concatenate  Mode=Multidimensional array  ConcatenateDimension=2
  wires:
  pos/1 -> State Writer1/1
  Vector Concatenate/1 -> State Writer/1
  Cos/1 -> Product/1
  vel/1 -> Product/2, Product1/2
  theta/1 -> Sin/1, Cos/1
  Product/1 -> Vector Concatenate/1
  Product1/1 -> Vector Concatenate/2
  Sin/1 -> Product1/1

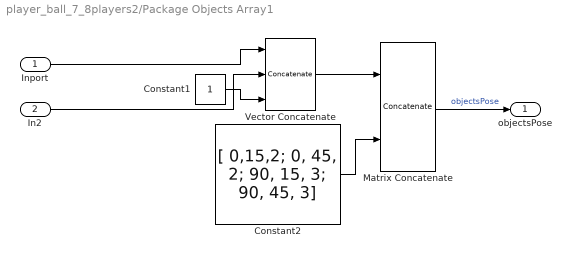
== system player_ball_7_8players2/Package Objects Array1 ==
  Inport : Inport
  In2 : Inport  Port=2
  Constant1 : Constant
  Constant2 : Constant  Value=[ 0,15,2; 0, 45, 2; 90, 15, 3; 90, 45, 3]
  Matrix Concatenate : Concatenate  Mode=Multidimensional array
  Vector Concatenate : Concatenate  NumInputs=3  Mode=Multidimensional array  ConcatenateDimension=2
  objectsPose : Outport  VectorParamsAs1DForOutWhenUnconnected=off
  wires:
  In2/1 -> Vector Concatenate/2
  Constant1/1 -> Vector Concatenate/3
  Inport/1 -> Vector Concatenate/1
  Constant2/1 -> Matrix Concatenate/2
  Matrix Concatenate/1 -> objectsPose/1  "objectsPose"
  Vector Concatenate/1 -> Matrix Concatenate/1

== matlab function player_ball_7_8players2/Zero Pad Detections2 ==
  data: u input size=[maxHits 3]; y output size=[maxHits 3]; maxHits parameter
function y = zeroPad(u,maxHits)
% Zero-pads object detections to work with arrays of buses

y = zeros(maxHits,3);
numElems = min(size(u,1),maxHits);
for idx = 1:numElems
   y(idx,1:3) = u(idx,1:3); 
end

== matlab function player_ball_7_8players2/Plot Soccer Field ==
function plotSoccerField
% Plots the soccer field once the figure window for the environment has
% been initialized

coder.extrinsic('evalin');
persistent hasPlotted
if isempty(hasPlotted)
    evalin('base','plotSoccerField');
    hasPlotted = true;
end

== matlab function player_ball_7_8players2/Zero Pad Detections3 ==
  data: u input size=[maxHits 3]; y output size=[maxHits 3]; maxHits parameter
function y = zeroPad(u,maxHits)
% Zero-pads object detections to work with arrays of buses

y = zeros(maxHits,3);
numElems = min(size(u,1),maxHits);
for idx = 1:numElems
   y(idx,1:3) = u(idx,1:3); 
end

== matlab function player_ball_7_8players2/ball ==
  data: u input; y output; ballHeld output; robotIdx output; ballHeld input; robotIdx input

function [y,ballHeld, robotIdx]= fcn(u,ballHeld,robotIdx)
a = u(1,:);
b = u(2,:);
c = u(3,:);
d = u(4,:);
e = u(5,:);
robotIdx =1;
if a(3) ==1
    y = a;


elseif b(3) ==1
    y = b;


elseif c(3)==1
    y=c;


elseif d(3)==1
    y=d;


else
    y = e;


end
if y(1)  <= 1.1
    ballHeld = 1;
    %robotIdx =1;
    %possession = robotIdx;

else
    ballHeld =0;
    %robotIdx =0;

end

== matlab function player_ball_7_8players2/Ball Dynamics ==
  data: ballPose output; ballHeld input; KickPower input; rPose_x input; rPose_y input; rPose_theta input
function ballPose  = fcn(ballHeld, KickPower,rPose_x, rPose_y, rPose_theta)
ballPose = [25 10];
if ballHeld == 1 
    ballPose = [rPose_x rPose_y] + (0.8 + 0.3)*[cos(rPose_theta) sin(rPose_theta)];

elseif KickPower >= 5.5 && ballHeld == 1
    %ballPose = KickPower*[rPose_x rPose_y] + (0.8 + 0.3)*[cos(rPose_theta) sin(rPose_theta)];
    ballHeld = 0
    ballPose = KickPower*[rPose_x rPose_y] + (0.8 + 0.3)*[cos(rPose_theta) sin(rPose_theta)];
    %if KickPower ~=0
    %    ballPose = KickPower*[rPose_x rPose_y] + (0.8 + 0.3)*[cos(rPose_theta) sin(rPose_theta)];
    %end

end

== matlab function player_ball_7_8players2/MATLAB Function ==
  data: u input; y output
function y = fcn(u)

if u > 3.15
    u = pi -(u - pi);
end

if u <-3.15
    u = pi + (u + pi);
end     

y = u;

== matlab function player_ball_7_8players2/idx3 goal_range_angles ==
  data: u input; goalRight_angle output; goalRange output; goalLeft_angle output; rPose_x input; rPose_y input
% function y = fcn(u)
% for i = 1:5
%     if u(i,3) == 1
%         a = u(i,:)
%     end
% end
% % b = u(2,:)
% % c = u(3,:)
% % d = u(4,:)
% % e = u(5,:)
% y = a;
% end
%two indexes are same. How to identify right and left angles
% for now randomly assigned the values
% goal range is minimum of the two 


function [goalRight_angle,goalRange, goalLeft_angle]= fcn(u,rPose_x, rPose_y)
goalRight_angle=0;
goalLeft_angle=0;
right_range = 0;
left_range =0;

x=0;
%if rPose_y1> 15 &&  rPose_y1< 45 && rPose_theta1 > 0
leftPolePose = [90 45];
rightPolePose = [90 15];
robotPose = [rPose_x rPose_y];
rightPole_dist = norm(rightPolePose - robotPose);
leftPole_dist = norm(leftPolePose - robotPose);
if rightPole_dist< leftPole_dist
    k=0;
    for i= 1:5
        if u(i,3) == 3 && k==0
            goalRight_angle = u(i,2);
            right_range = u(i,1);
            k = k+1;
        elseif u(i,3) ==3 && k==1
            goalLeft_angle = u(i,2);
            left_range = u(i,1);
            k =0;

        end
    end
else
    k=0;
    for i= 1:5
        if u(i,3) == 3 && k==0
            goalLeft_angle = u(i,2);
            left_range = u(i,1);
            k = k+1;
        elseif u(i,3) ==3 && k==1
            goalRight_angle = u(i,2);
            right_range = u(i,1);
            k =0;

        end
    end
end

if right_range < left_range
    goalRange = right_range;
else
    goalRange = left_range;
end
